simulink model "RASS"  (R2023b)
settings: Solver=FixedStepAuto  StartTime=0.0  StopTime=10000  FixedStep=0.001  RelTol=1e-3
values from neighbouring files (symbols this model uses):
  A = [0 0 1 0 0 0 0 0 1 0 -50 500 ... (25 elements, 5x5)]    [RASS.mat]    (also in RASS_parameters.m = [0, 1, 0, 0; -k_s/m_s, -c_s/m_s, k_s/m_s, c_s/m_s; 0, 0, 0, )
  B = [0.0025 -0.025 0 0 0]    [RASS.mat]    (also in RASS_parameters.m = [0, 0; 0, 1/m_s; 0, 0; 1/m_u, 1/m_u])
  C = [0 0 0 0 0 0 -50 1 0 50 -1 1 ... (15 elements, 3x5)]    [RASS.mat]    (also in RASS_parameters.m = [-k_s/m_s, -c_s/m_s, k_s/m_s, c_s/m_s; 0, 1, 0, 0; 0, 0, 0, )
  D = [0.0025 0 0]    [RASS.mat]    (also in RASS_parameters.m = [0, 1/m_s; 0, 0; 0, 0])
  H = [0 0 0 0 0.0224794071393]    [RASS.mat]
libraries: slpidlib x1
settings Model: Creator=Mikael  LastModifiedBy=Mikael

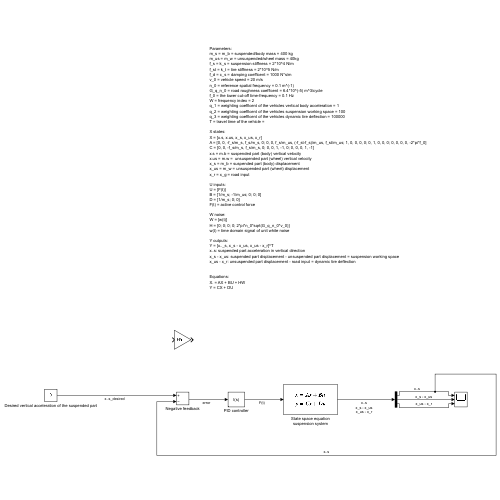
[thumbnail: Simulink's stored preview of the top-level diagram]
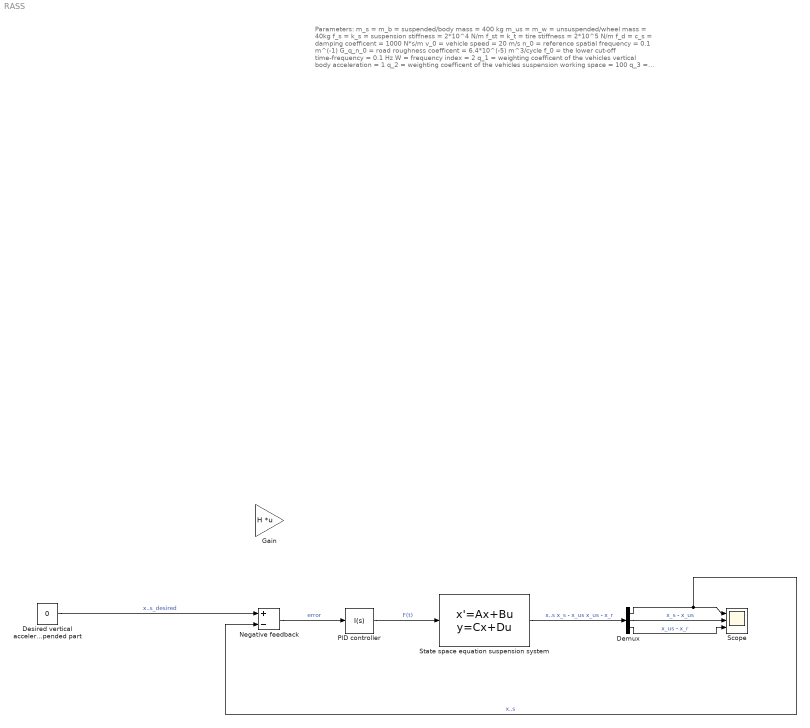
== system RASS ==
  note: Parameters:
      | m_s = m_b = suspended/body mass = 400 kg
      | m_us = m_w = unsuspended/wheel mass = 40kg
      | f_s = k_s = suspension stiffness = 2*10^4 N/m
      | f_st = k_t = tire stiffness = 2*10^5 N/m
      | f_d = c_s = damping coefficent = 1000 N*s/m
      | v_0 = vehicle speed = 20 m/s
      | n_0 = reference spatial frequency = 0.1 m^(-1)
      | G_q_n_0 = road roughness coefficent = 6.4*10^(-5) m^3/cycle
      | f_0 = the lower cut-off time-frequency = 0.1 Hz
      | W = frequency index = 2
      | q_1 = weighting coefficent of the vehicles vertical body acceleration = 1
      | q_2 = weighting coefficent of the vehicles suspension working space = 100
      | q_3 = weighting coefficent of the vehicles dynamic tire deflection = 100000
      | T = travel time of the vehicle =
      |
      | X states:
      | X = [x.s, x.us, x_s, x_us, x_r]
      | A = [0, 0, -f_s/m_s, f_s/m_s, 0; 0, 0, f_s/m_us, (-f_st-f_s)/m_us, f_st/m_us; 1, 0, 0, 0, 0; 0, 1, 0, 0, 0; 0, 0, 0, 0, -2*pi*f_0]
      | C = [0, 0, -f_s/m_s, f_s/m_s, 0; 0, 0, 1, -1, 0; 0, 0, 0, 1, -1]
      | x.s = m.b = suspended part (body) vertical velocity
      | x.us = m.w = unsuspended part (wheel) vertical velocity
      | x_s = m_b = suspended part (body) displacement
      | x_us = m_w = unsuspended part (wheel) displacement
      | x_r = x_g = road input
      |
      | U inputs:
      | U = [F(t)]
      | B = [1/m_s; -1/m_us; 0; 0; 0]
      | D = [1/m_s; 0; 0]
      | F(t) = active control force
      |
      | W noise:
      | W = [w(t)]
      | H = [0; 0; 0; 0; 2*pi*n_0*sqrt(G_q_n_0*v_0)]
      | w(t) = time domain signal of unit white noise
      |
      | Y outputs:
      | Y = [x.._s, x_s - x_us, x_us - x_r]^T
      | x..s: suspended part acceleration in vertical direction
      | x_s - x_us: suspended part displacement - unsuspended part displacement = suspension working space
      | x_us - x_r: unsuspended part displacement - road input = dynamic tire deflection
      |
      | Equations:
      | X. = AX + BU + HW
      | Y = CX + DU
  Demux : Demux  Outputs=3
  Desired vertical acceleration of the suspended part : Constant  Value=0
  Gain : Gain  Gain=H  Multiplication=Matrix(K*u)
  Negative feedback : Sum  Inputs=+-
  PID controller : slpidlib/PID Controller  Controller=I  Form=Parallel  TimeDomain=Continuous-time  UseExternalTs=off  SampleTime=-1  IntegratorMethod=Forward Euler  FilterMethod=Forward Euler  ControllerParametersSource=internal  P=0  I=172.352408008124  UseKiTs=off  D=0  N=100  UseFilter=on  TunerSelectOption=Transfer Function Based (PID Tuner App)  InitialConditionSource=internal  InitialConditionForIntegrator=0  InitialConditionForFilter=0  DifferentiatorICPrevScaledInput=0  ExternalReset=none  TrackingMode=off  Kt=1  LimitOutput=off  SatLimitsSource=internal  UpperSaturationLimit=inf  LowerSaturationLimit=-inf  LinearizeAsGain=on  AntiWindupMode=none  Kb=1  LimitIntegrator=off  UpperIntegratorSaturationLimit=inf  LowerIntegratorSaturationLimit=-inf  POutMin=[]  POutMax=[]  IOutMin=[]  IOutMax=[]  DOutMin=[]  DOutMax=[]  NOutMin=[]  NOutMax=[]  SumOutMin=[]  SumOutMax=[]  SaturationOutMin=[]  SaturationOutMax=[]  PParamMin=[]  PParamMax=[]  IParamMin=[]  IParamMax=[]  DParamMin=[]  DParamMax=[]  NParamMin=[]  NParamMax=[]  KbParamMin=[]  KbParamMax=[]  KtParamMin=[]  KtParamMax=[]  KbOutMin=[]  KbOutMax=[]  KtOutMin=[]  KtOutMax=[]  IntegratorOutMin=[]  IntegratorOutMax=[]  FilterOutMin=[]  FilterOutMax=[]  SumI1OutMin=[]  SumI1OutMax=[]  SumI2OutMin=[]  SumI2OutMax=[]  SumI3OutMin=[]  SumI3OutMax=[]  SumI4OutMin=[]  SumI4OutMax=[]  SumDOutMin=[]  SumDOutMax=[]  DifferentiatorOutMin=[]  DifferentiatorOutMax=[]  FilterDiffOutCoefMin=[]  FilterDiffOutCoefMax=[]  ReciprocalOutMin=[]  ReciprocalOutMax=[]  SumDenOutMin=[]  SumDenOutMax=[]  SumNumOutMin=[]  SumNumOutMax=[]  DivideOutMin=[]  DivideOutMax=[]  UdiffTsProdOutMin=[]  UdiffTsProdOutMax=[]  NTsProdOutMin=[]  NTsProdOutMax=[]  UintegralTsProdOutMin=[]  UintegralTsProdOutMax=[]  UngainTsProdOutMin=[]  UngainTsProdOutMax=[]  ClampingZeroOutDataTypeStr=Inherit: Inherit via back propagation  ClampingZeroOutMin=[]  ClampingZeroOutMax=[]  FilterDenConstantOutDataTypeStr=Inherit: Inherit via back propagation  FilterDenConstantOutMin=[]  FilterDenConstantOutMax=[]  PCopyOutDataTypeStr=Inherit: Inherit via back propagation  PCopyOutMin=[]  PCopyOutMax=[]  NCopyOutDataTypeStr=Inherit: Inherit via back propagation  NCopyOutMin=[]  NCopyOutMax=[]  IntegratorContinuousStateAttributes=''  IntegratorStateMustResolveToSignalObject=off  IntegratorRTWStateStorageClass=Auto  FilterContinuousStateAttributes=''  FilterStateMustResolveToSignalObject=off  FilterRTWStateStorageClass=Auto  ParallelPVariant=Disabled  IdealPVariant=Disabled  IVariant=InternalParameters  DVariant=Disabled  IntegratorVariant=Continuous  SatVariant=Disabled  AWVariant=Passthrough  PCopyVariant=Disabled  TRVariant=Disabled  FdbkBlocksVariant=Forward  IdealPFdbkVariant=Disabled  SatFdbkVariant=Disabled  DerivativeFilterVariant=Disabled  NVariant=Disabled  NCopyVariant=Disabled_SignalSpec  FilterICVariant=Disabled  IntegratorICVariant=InternalICs  ExternalResetVariant=Disabled  TRSumVariant=Passthrough  SumFdbkVariant=Disabled  SumVariant=Passthrough_I  TsampFilterVariant=InternalTs  TsampNgainVariant=Passthrough  TsampIntegralVariant=Disabled_SignalSpec  ExternalSaturationOutDataTypeStr=Inherit: Same as second input
  Scope : Scope  NumInputPorts=3
  State space equation suspension system : StateSpace  A=A  B=B  C=C  D=D  InitialCondition=0
  wires:
  State space equation suspension system/1 -> Demux/1  "x..s x_s - x_us x_us - x_r"
  PID controller/1 -> State space equation suspension system/1  "F(t)"
  Demux/2 -> Scope/2  "x_s - x_us"
  Demux/1 -> Scope/1, Negative feedback/2  "x..s"
  Demux/3 -> Scope/3  "x_us - x_r"
  Negative feedback/1 -> PID controller/1  "error"
  Desired vertical acceleration of the suspended part/1 -> Negative feedback/1  "x..s_desired"
